simulink model "gm_uz_Deadbeat"  (R2022a)
settings: Solver=FixedStepDiscrete  StartTime=0.0  StopTime=10.0  RelTol=1e-3
settings Model: Creator=go98noz  LastModifiedBy=go98noz
settings SolverCC: AlgebraicLoopSolver=TrustRegion
settings DataIOCC: LimitDataPoints=on  SaveOutput=off  SaveTime=off
settings OptimizationCC: BlockReduction=off  ConditionallyExecuteInputs=off  DefaultParameterBehavior=Inlined  InheritOutputTypeSmallerThanSingle=on  LifeSpan=inf
settings DebuggingCC: AlgebraicLoopMsg=error  InheritedTsInSrcMsg=none  SingleTaskRateTransMsg=error  UnconnectedInputMsg=warning  UnconnectedOutputMsg=warning  UnconnectedLineMsg=warning  AllowSymbolicDim=off  StrictBusMsg=ErrorOnBusTreatedAsVector  SFUnexpectedBacktrackingDiag=warning  SFNoUnconditionalDefaultTransitionDiag=warning  SFExecutionAtInitializationDiag=none  SFMachineParentedDataDiag=warning  ArithmeticOperatorsInVariantConditions=warning
settings HardwareCC: ProdBitPerPointer=32  ProdBitPerSizeT=32  ProdBitPerPtrDiffT=32  ProdLargestAtomicFloat=None  ProdIntDivRoundTo=Undefined  ProdEndianess=Unspecified  ProdWordSize=32  ProdHWDeviceType=ASIC/FPGA->ASIC/FPGA  ProdEqTarget=off
settings SFSimCC: SimUseLocalCustomCode=off  CustomCodeUndefinedFunction=UseInterfaceOnly
settings RTWCC: RTWUseLocalCustomCode=off
settings CodeAppCC: StateflowObjectComments=on
settings GRTTargetCC: TargetLangStandard=C89/C90 (ANSI)
settings ConfigComp: CovScope=ReferencedModels  CovMetricSettings=dw  CovSaveCumulativeToWorkspaceVar=on  CovSaveSingleToWorkspaceVar=on  CovExternalEMLEnable=off  CovSFcnEnable=off

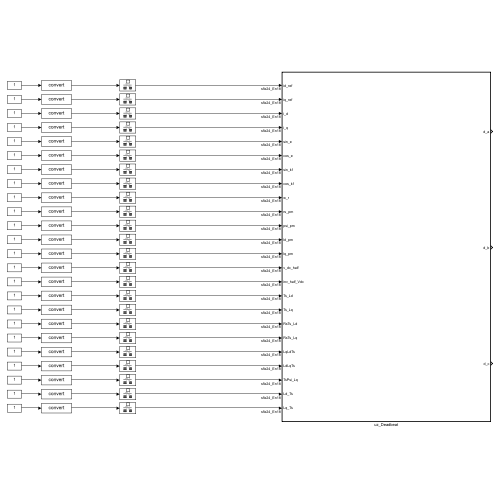
[thumbnail: Simulink's stored preview of the top-level diagram]
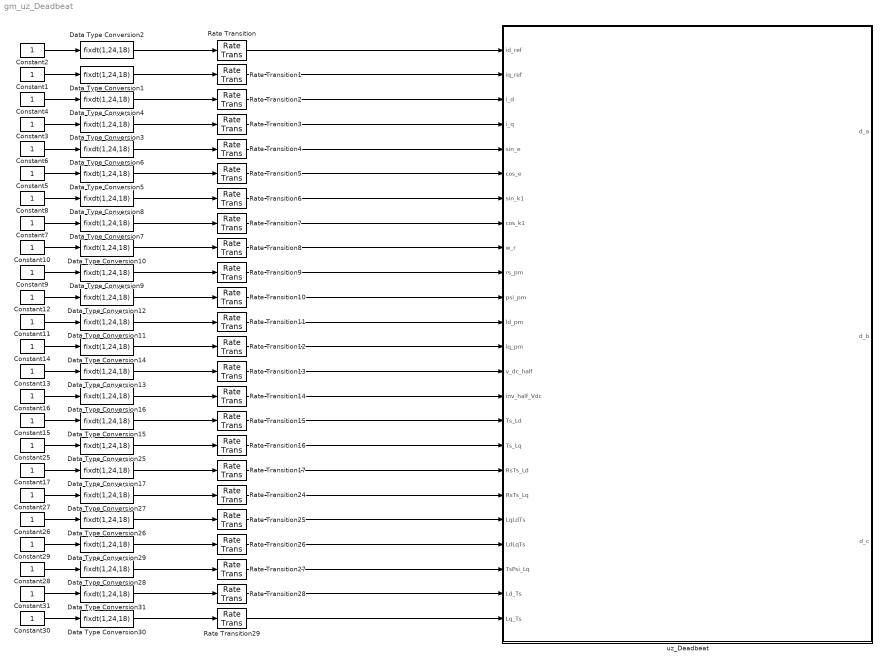
== system gm_uz_Deadbeat ==
  Constant{1..17,25..31} (24 alike) : Constant
  Data Type Conversion{1..17,25..31} (24 alike) : DataTypeConversion  OutDataTypeStr=fixdt(1,24,18)  SaturateOnIntegerOverflow=off  RndMeth=Floor
  Rate Transition{,1..17,24..29} (24 alike) : RateTransition  OutPortSampleTime=1/100e6
  uz_Deadbeat : Subsystem  TreatAsAtomicUnit=on
  wires:
  Rate Transition29/1 -> uz_Deadbeat/24(Lq_Ts)
  Rate Transition28/1 -> uz_Deadbeat/23(Ld_Ts)
  Rate Transition27/1 -> uz_Deadbeat/22(TsPsi_Lq)
  Rate Transition26/1 -> uz_Deadbeat/21(LdLqTs)
  Rate Transition25/1 -> uz_Deadbeat/20(LqLdTs)
  Rate Transition24/1 -> uz_Deadbeat/19(RsTs_Lq)
  Rate Transition17/1 -> uz_Deadbeat/18(RsTs_Ld)
  Rate Transition16/1 -> uz_Deadbeat/17(Ts_Lq)
  Rate Transition15/1 -> uz_Deadbeat/16(Ts_Ld)
  Rate Transition14/1 -> uz_Deadbeat/15(inv_half_Vdc)
  Rate Transition13/1 -> uz_Deadbeat/14(v_dc_half)
  Rate Transition12/1 -> uz_Deadbeat/13(lq_pm)
  Rate Transition11/1 -> uz_Deadbeat/12(ld_pm)
  Rate Transition10/1 -> uz_Deadbeat/11(psi_pm)
  Rate Transition9/1 -> uz_Deadbeat/10(rs_pm)
  Rate Transition8/1 -> uz_Deadbeat/9(w_r)
  Rate Transition7/1 -> uz_Deadbeat/8(cos_k1)
  Rate Transition6/1 -> uz_Deadbeat/7(sin_k1)
  Rate Transition5/1 -> uz_Deadbeat/6(cos_e)
  Rate Transition4/1 -> uz_Deadbeat/5(sin_e)
  Rate Transition3/1 -> uz_Deadbeat/4(i_q)
  Rate Transition2/1 -> uz_Deadbeat/3(i_d)
  Data Type Conversion17/1 -> Rate Transition17/1
  Constant17/1 -> Data Type Conversion17/1
  Constant25/1 -> Data Type Conversion25/1
  Data Type Conversion25/1 -> Rate Transition16/1
  Data Type Conversion27/1 -> Rate Transition24/1
  Constant27/1 -> Data Type Conversion27/1
  Constant26/1 -> Data Type Conversion26/1
  Data Type Conversion26/1 -> Rate Transition25/1
  Data Type Conversion30/1 -> Rate Transition29/1
  Constant30/1 -> Data Type Conversion30/1
  Constant31/1 -> Data Type Conversion31/1
  Data Type Conversion31/1 -> Rate Transition28/1
  Data Type Conversion29/1 -> Rate Transition26/1
  Constant29/1 -> Data Type Conversion29/1
  Constant28/1 -> Data Type Conversion28/1
  Data Type Conversion28/1 -> Rate Transition27/1
  Data Type Conversion9/1 -> Rate Transition9/1
  Constant9/1 -> Data Type Conversion9/1
  Constant10/1 -> Data Type Conversion10/1
  Data Type Conversion10/1 -> Rate Transition8/1
  Data Type Conversion12/1 -> Rate Transition10/1
  Constant12/1 -> Data Type Conversion12/1
  Constant11/1 -> Data Type Conversion11/1
  Data Type Conversion11/1 -> Rate Transition11/1
  Data Type Conversion15/1 -> Rate Transition15/1
  Constant15/1 -> Data Type Conversion15/1
  Constant16/1 -> Data Type Conversion16/1
  Data Type Conversion16/1 -> Rate Transition14/1
  Data Type Conversion14/1 -> Rate Transition12/1
  Constant14/1 -> Data Type Conversion14/1
  Constant13/1 -> Data Type Conversion13/1
  Data Type Conversion13/1 -> Rate Transition13/1
  Data Type Conversion5/1 -> Rate Transition5/1
  Constant5/1 -> Data Type Conversion5/1
  Constant6/1 -> Data Type Conversion6/1
  Data Type Conversion6/1 -> Rate Transition4/1
  Data Type Conversion8/1 -> Rate Transition6/1
  Constant8/1 -> Data Type Conversion8/1
  Constant7/1 -> Data Type Conversion7/1
  Data Type Conversion7/1 -> Rate Transition7/1
  Data Type Conversion3/1 -> Rate Transition3/1
  Constant3/1 -> Data Type Conversion3/1
  Constant4/1 -> Data Type Conversion4/1
  Data Type Conversion4/1 -> Rate Transition2/1
  Data Type Conversion2/1 -> Rate Transition/1
  Constant2/1 -> Data Type Conversion2/1
  Constant1/1 -> Data Type Conversion1/1
  Data Type Conversion1/1 -> Rate Transition1/1
  Rate Transition1/1 -> uz_Deadbeat/2(iq_ref)
  Rate Transition/1 -> uz_Deadbeat/1(id_ref)

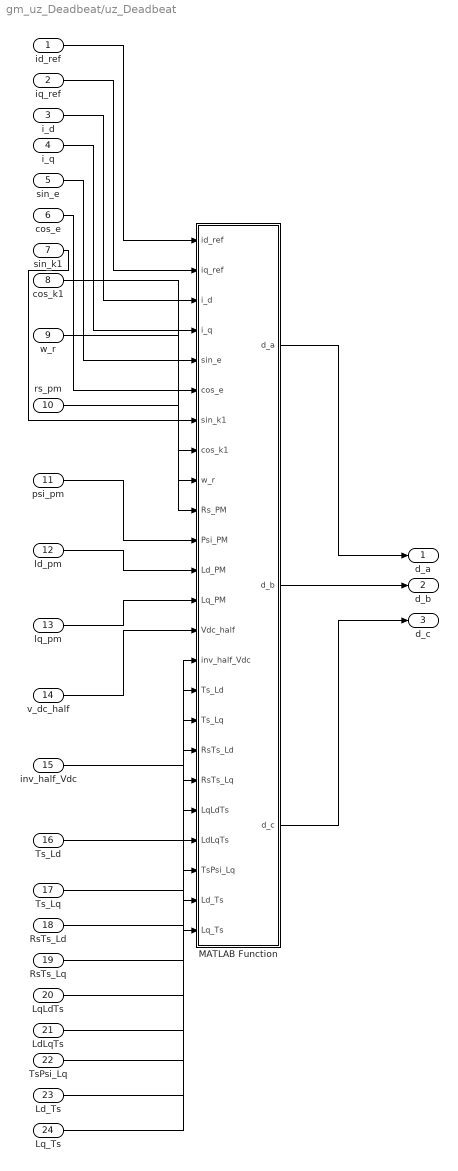
== system gm_uz_Deadbeat/uz_Deadbeat ==
  id_ref : Inport  OutDataTypeStr=fixdt(1, 24, 18)  PortDimensions=1  SampleTime=1e-08
  iq_ref : Inport  Port=2  OutDataTypeStr=fixdt(1, 24, 18)  PortDimensions=1  SampleTime=1e-08
  i_d : Inport  Port=3  OutDataTypeStr=fixdt(1, 24, 18)  PortDimensions=1  SampleTime=1e-08
  i_q : Inport  Port=4  OutDataTypeStr=fixdt(1, 24, 18)  PortDimensions=1  SampleTime=1e-08
  sin_e : Inport  Port=5  OutDataTypeStr=fixdt(1, 24, 18)  PortDimensions=1  SampleTime=1e-08
  cos_e : Inport  Port=6  OutDataTypeStr=fixdt(1, 24, 18)  PortDimensions=1  SampleTime=1e-08
  sin_k1 : Inport  Port=7  OutDataTypeStr=fixdt(1, 24, 18)  PortDimensions=1  SampleTime=1e-08
  cos_k1 : Inport  Port=8  OutDataTypeStr=fixdt(1, 24, 18)  PortDimensions=1  SampleTime=1e-08
  w_r : Inport  Port=9  OutDataTypeStr=fixdt(1, 24, 18)  PortDimensions=1  SampleTime=1e-08
  rs_pm : Inport  Port=10  OutDataTypeStr=fixdt(1, 24, 18)  PortDimensions=1  SampleTime=1e-08
  psi_pm : Inport  Port=11  OutDataTypeStr=fixdt(1, 24, 18)  PortDimensions=1  SampleTime=1e-08
  ld_pm : Inport  Port=12  OutDataTypeStr=fixdt(1, 24, 18)  PortDimensions=1  SampleTime=1e-08
  lq_pm : Inport  Port=13  OutDataTypeStr=fixdt(1, 24, 18)  PortDimensions=1  SampleTime=1e-08
  v_dc_half : Inport  Port=14  OutDataTypeStr=fixdt(1, 24, 18)  PortDimensions=1  SampleTime=1e-08
  inv_half_Vdc : Inport  Port=15  OutDataTypeStr=fixdt(1, 24, 18)  PortDimensions=1  SampleTime=1e-08
  Ts_Ld : Inport  Port=16  OutDataTypeStr=fixdt(1, 24, 18)  PortDimensions=1  SampleTime=1e-08
  Ts_Lq : Inport  Port=17  OutDataTypeStr=fixdt(1, 24, 18)  PortDimensions=1  SampleTime=1e-08
  RsTs_Ld : Inport  Port=18  OutDataTypeStr=fixdt(1, 24, 18)  PortDimensions=1  SampleTime=1e-08
  RsTs_Lq : Inport  Port=19  OutDataTypeStr=fixdt(1, 24, 18)  PortDimensions=1  SampleTime=1e-08
  LqLdTs : Inport  Port=20  OutDataTypeStr=fixdt(1, 24, 18)  PortDimensions=1  SampleTime=1e-08
  LdLqTs : Inport  Port=21  OutDataTypeStr=fixdt(1, 24, 18)  PortDimensions=1  SampleTime=1e-08
  TsPsi_Lq : Inport  Port=22  OutDataTypeStr=fixdt(1, 24, 18)  PortDimensions=1  SampleTime=1e-08
  Ld_Ts : Inport  Port=23  OutDataTypeStr=fixdt(1, 24, 18)  PortDimensions=1  SampleTime=1e-08
  Lq_Ts : Inport  Port=24  OutDataTypeStr=fixdt(1, 24, 18)  PortDimensions=1  SampleTime=1e-08
  MATLAB Function : Subsystem
  d_a : Outport  SampleTime=1e-08  VectorParamsAs1DForOutWhenUnconnected=off
  d_b : Outport  Port=2  SampleTime=1e-08  VectorParamsAs1DForOutWhenUnconnected=off
  d_c : Outport  Port=3  SampleTime=1e-08  VectorParamsAs1DForOutWhenUnconnected=off
  wires:
  id_ref/1 -> MATLAB Function/1(id_ref)
  iq_ref/1 -> MATLAB Function/2(iq_ref)
  i_d/1 -> MATLAB Function/3(i_d)
  i_q/1 -> MATLAB Function/4(i_q)
  sin_e/1 -> MATLAB Function/5(sin_e)
  cos_e/1 -> MATLAB Function/6(cos_e)
  sin_k1/1 -> MATLAB Function/7(sin_k1)
  cos_k1/1 -> MATLAB Function/8(cos_k1)
  w_r/1 -> MATLAB Function/9(w_r)
  rs_pm/1 -> MATLAB Function/10(Rs_PM)
  psi_pm/1 -> MATLAB Function/11(Psi_PM)
  ld_pm/1 -> MATLAB Function/12(Ld_PM)
  lq_pm/1 -> MATLAB Function/13(Lq_PM)
  v_dc_half/1 -> MATLAB Function/14(Vdc_half)
  inv_half_Vdc/1 -> MATLAB Function/15(inv_half_Vdc)
  Ts_Ld/1 -> MATLAB Function/16(Ts_Ld)
  Ts_Lq/1 -> MATLAB Function/17(Ts_Lq)
  RsTs_Ld/1 -> MATLAB Function/18(RsTs_Ld)
  RsTs_Lq/1 -> MATLAB Function/19(RsTs_Lq)
  LqLdTs/1 -> MATLAB Function/20(LqLdTs)
  LdLqTs/1 -> MATLAB Function/21(LdLqTs)
  TsPsi_Lq/1 -> MATLAB Function/22(TsPsi_Lq)
  Ld_Ts/1 -> MATLAB Function/23(Ld_Ts)
  Lq_Ts/1 -> MATLAB Function/24(Lq_Ts)
  MATLAB Function/1(d_a) -> d_a/1
  MATLAB Function/2(d_b) -> d_b/1
  MATLAB Function/3(d_c) -> d_c/1

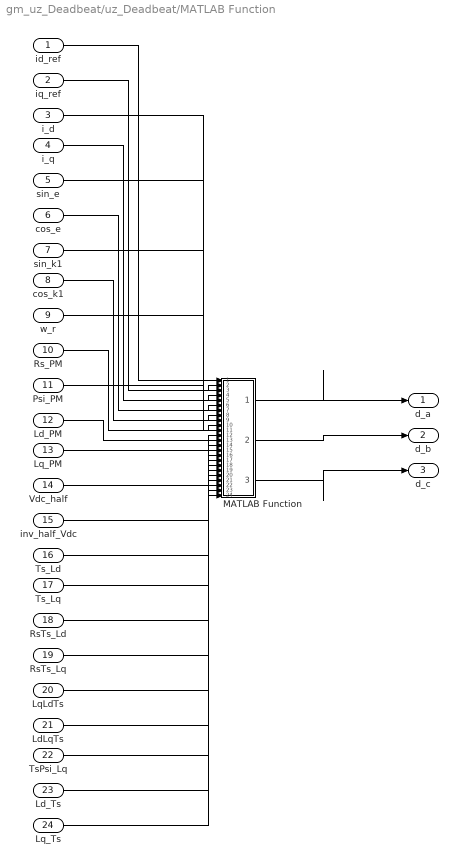
== system gm_uz_Deadbeat/uz_Deadbeat/MATLAB Function ==
  id_ref : Inport  OutDataTypeStr=fixdt(1, 24, 18)  PortDimensions=1  SampleTime=1e-08
  iq_ref : Inport  Port=2  OutDataTypeStr=fixdt(1, 24, 18)  PortDimensions=1  SampleTime=1e-08
  i_d : Inport  Port=3  OutDataTypeStr=fixdt(1, 24, 18)  PortDimensions=1  SampleTime=1e-08
  i_q : Inport  Port=4  OutDataTypeStr=fixdt(1, 24, 18)  PortDimensions=1  SampleTime=1e-08
  sin_e : Inport  Port=5  OutDataTypeStr=fixdt(1, 24, 18)  PortDimensions=1  SampleTime=1e-08
  cos_e : Inport  Port=6  OutDataTypeStr=fixdt(1, 24, 18)  PortDimensions=1  SampleTime=1e-08
  sin_k1 : Inport  Port=7  OutDataTypeStr=fixdt(1, 24, 18)  PortDimensions=1  SampleTime=1e-08
  cos_k1 : Inport  Port=8  OutDataTypeStr=fixdt(1, 24, 18)  PortDimensions=1  SampleTime=1e-08
  w_r : Inport  Port=9  OutDataTypeStr=fixdt(1, 24, 18)  PortDimensions=1  SampleTime=1e-08
  Rs_PM : Inport  Port=10  OutDataTypeStr=fixdt(1, 24, 18)  PortDimensions=1  SampleTime=1e-08
  Psi_PM : Inport  Port=11  OutDataTypeStr=fixdt(1, 24, 18)  PortDimensions=1  SampleTime=1e-08
  Ld_PM : Inport  Port=12  OutDataTypeStr=fixdt(1, 24, 18)  PortDimensions=1  SampleTime=1e-08
  Lq_PM : Inport  Port=13  OutDataTypeStr=fixdt(1, 24, 18)  PortDimensions=1  SampleTime=1e-08
  Vdc_half : Inport  Port=14  OutDataTypeStr=fixdt(1, 24, 18)  PortDimensions=1  SampleTime=1e-08
  inv_half_Vdc : Inport  Port=15  OutDataTypeStr=fixdt(1, 24, 18)  PortDimensions=1  SampleTime=1e-08
  Ts_Ld : Inport  Port=16  OutDataTypeStr=fixdt(1, 24, 18)  PortDimensions=1  SampleTime=1e-08
  Ts_Lq : Inport  Port=17  OutDataTypeStr=fixdt(1, 24, 18)  PortDimensions=1  SampleTime=1e-08
  RsTs_Ld : Inport  Port=18  OutDataTypeStr=fixdt(1, 24, 18)  PortDimensions=1  SampleTime=1e-08
  RsTs_Lq : Inport  Port=19  OutDataTypeStr=fixdt(1, 24, 18)  PortDimensions=1  SampleTime=1e-08
  LqLdTs : Inport  Port=20  OutDataTypeStr=fixdt(1, 24, 18)  PortDimensions=1  SampleTime=1e-08
  LdLqTs : Inport  Port=21  OutDataTypeStr=fixdt(1, 24, 18)  PortDimensions=1  SampleTime=1e-08
  TsPsi_Lq : Inport  Port=22  OutDataTypeStr=fixdt(1, 24, 18)  PortDimensions=1  SampleTime=1e-08
  Ld_Ts : Inport  Port=23  OutDataTypeStr=fixdt(1, 24, 18)  PortDimensions=1  SampleTime=1e-08
  Lq_Ts : Inport  Port=24  OutDataTypeStr=fixdt(1, 24, 18)  PortDimensions=1  SampleTime=1e-08
  MATLAB Function : MATLAB Function  TreatAsAtomicUnit=on
  d_a : Outport  SampleTime=1e-08  VectorParamsAs1DForOutWhenUnconnected=off
  d_b : Outport  Port=2  SampleTime=1e-08
  d_c : Outport  Port=3  SampleTime=1e-08
  wires:
  id_ref/1 -> MATLAB Function/1(id_ref)
  iq_ref/1 -> MATLAB Function/2(iq_ref)
  i_d/1 -> MATLAB Function/3(i_d)
  i_q/1 -> MATLAB Function/4(i_q)
  sin_e/1 -> MATLAB Function/5(sin_e)
  cos_e/1 -> MATLAB Function/6(cos_e)
  sin_k1/1 -> MATLAB Function/7(sin_k1)
  cos_k1/1 -> MATLAB Function/8(cos_k1)
  w_r/1 -> MATLAB Function/9(w_r)
  Rs_PM/1 -> MATLAB Function/10(Rs_PM)
  Psi_PM/1 -> MATLAB Function/11(Psi_PM)
  Ld_PM/1 -> MATLAB Function/12(Ld_PM)
  Lq_PM/1 -> MATLAB Function/13(Lq_PM)
  Vdc_half/1 -> MATLAB Function/14(Vdc_half)
  inv_half_Vdc/1 -> MATLAB Function/15(inv_half_Vdc)
  Ts_Ld/1 -> MATLAB Function/16(Ts_Ld)
  Ts_Lq/1 -> MATLAB Function/17(Ts_Lq)
  RsTs_Ld/1 -> MATLAB Function/18(RsTs_Ld)
  RsTs_Lq/1 -> MATLAB Function/19(RsTs_Lq)
  LqLdTs/1 -> MATLAB Function/20(LqLdTs)
  LdLqTs/1 -> MATLAB Function/21(LdLqTs)
  TsPsi_Lq/1 -> MATLAB Function/22(TsPsi_Lq)
  Ld_Ts/1 -> MATLAB Function/23(Ld_Ts)
  Lq_Ts/1 -> MATLAB Function/24(Lq_Ts)
  MATLAB Function/1(d_a) -> d_a/1
  MATLAB Function/2(d_b) -> d_b/1
  MATLAB Function/3(d_c) -> d_c/1

== matlab function gm_uz_Deadbeat/uz_Deadbeat/MATLAB Function/MATLAB Function ==
  settings: fimath=fimath('RoundingMethod', 'Floor','OverflowAction', 'Wrap','ProductMode', 'FullPrecision', 'SumMode', 'FullPrecision')
  data: id_ref input; d_a output fixdt(0,16,15); iq_ref input; i_d input; i_q input; sin_e input; cos_e input; sin_k1 input; cos_k1 input; w_r input; Rs_PM input; Psi_PM input; Ld_PM input; Lq_PM input; Vdc_half input; inv_half_Vdc input; Ts_Ld input; d_b output fixdt(0,16,15); d_c output fixdt(0,16,15); Ts_Lq input; RsTs_Ld input; RsTs_Lq input; LqLdTs input; LdLqTs input; TsPsi_Lq input; Ld_Ts input; Lq_Ts input
function [d_a, d_b, d_c] = DB_PWM( ...
    id_ref, iq_ref, i_d, i_q, ...
    sin_e, cos_e, sin_k1, cos_k1, ...
    w_r, Rs_PM, Psi_PM, Ld_PM, Lq_PM, ...
    Vdc_half, inv_half_Vdc, ...
    Ts_Ld, Ts_Lq, RsTs_Ld, RsTs_Lq, ...
    LqLdTs, LdLqTs, TsPsi_Lq, ...
    Ld_Ts, Lq_Ts)

%#codegen

Tcur  = numerictype(1,24,16);
Tvol  = numerictype(1,24,10);
Tmod  = numerictype(1,18,16);
Tcoef = numerictype(1,24,18);
Ttrig = numerictype(1,18,16);
Tout  = numerictype(0,16,15);

F = fimath( ...
    'RoundingMethod','Nearest', ...
    'OverflowAction','Saturate', ...
    'ProductMode','SpecifyPrecision', ...
    'ProductWordLength',32, ...
    'ProductFractionLength',20, ...
    'SumMode','SpecifyPrecision', ...
    'SumWordLength',32, ...
    'SumFractionLength',20);

id_ref = fi(id_ref, Tcur, F);
iq_ref = fi(iq_ref, Tcur, F);
i_d    = fi(i_d,    Tcur, F);
i_q    = fi(i_q,    Tcur, F);

sin_e  = fi(sin_e,  Ttrig, F);
cos_e  = fi(cos_e,  Ttrig, F);
sin_k1 = fi(sin_k1, Ttrig, F);
cos_k1 = fi(cos_k1, Ttrig, F);

w_r          = fi(w_r,          Tcoef, F);
Rs_PM        = fi(Rs_PM,        Tcoef, F);
Psi_PM       = fi(Psi_PM,       Tcoef, F);
Ld_PM        = fi(Ld_PM,        Tcoef, F);
Lq_PM        = fi(Lq_PM,        Tcoef, F);
Vdc_half     = fi(Vdc_half,     Tcoef, F);
inv_half_Vdc = fi(inv_half_Vdc, Tcoef, F);

Ts_Ld     = fi(Ts_Ld,     Tcoef, F);
Ts_Lq     = fi(Ts_Lq,     Tcoef, F);
RsTs_Ld   = fi(RsTs_Ld,   Tcoef, F);
RsTs_Lq   = fi(RsTs_Lq,   Tcoef, F);
LqLdTs    = fi(LqLdTs,    Tcoef, F);
LdLqTs    = fi(LdLqTs,    Tcoef, F);
TsPsi_Lq  = fi(TsPsi_Lq,  Tcoef, F);
Ld_Ts     = fi(Ld_Ts,     Tcoef, F);
Lq_Ts     = fi(Lq_Ts,     Tcoef, F);

zero_mod = fi(0, Tmod, F);

persistent u_a0 u_b0 u_c0;
if isempty(u_a0)
    u_a0 = zero_mod;
    u_b0 = zero_mod;
    u_c0 = zero_mod;
end

[u_alpha0, u_beta0] = T_C(u_a0, u_b0, u_c0, F);

[u_d0, u_q0] = T_P(u_alpha0, u_beta0, sin_e, cos_e, F);

v_d0 = fi(u_d0 * Vdc_half, Tvol, F);
v_q0 = fi(u_q0 * Vdc_half, Tvol, F);

one_coef = fi(1, Tcoef, F);

term_id1 = fi(Ts_Ld * v_d0, Tcur, F);
term_id2 = fi(fi(one_coef - RsTs_Ld, Tcoef, F) * i_d, Tcur, F);
term_id3 = fi(fi(LqLdTs * w_r, Tcoef, F) * i_q, Tcur, F);

id_k = fi(term_id1 + term_id2 + term_id3, Tcur, F);

term_iq1 = fi(Ts_Lq * v_q0, Tcur, F);
term_iq2 = fi(fi(one_coef - RsTs_Lq, Tcoef, F) * i_q, Tcur, F);
term_iq3 = fi(fi(LdLqTs * w_r, Tcoef, F) * i_d, Tcur, F);
term_iq4 = fi(TsPsi_Lq * w_r, Tcur, F);

iq_k = fi(term_iq1 + term_iq2 - term_iq3 - term_iq4, Tcur, F);

err_d = fi(id_ref - id_k, Tcur, F);
err_q = fi(iq_ref - iq_k, Tcur, F);

term_vd1 = fi(Ld_Ts * err_d, Tvol, F);
term_vd2 = fi(Rs_PM * id_k,  Tvol, F);
term_vd3 = fi(fi(Lq_PM * w_r, Tcoef, F) * iq_k, Tvol, F);

vd_ref = fi(term_vd1 + term_vd2 - term_vd3, Tvol, F);

term_vq1 = fi(Lq_Ts * err_q, Tvol, F);
term_vq2 = fi(Rs_PM * iq_k,  Tvol, F);
term_vq3 = fi(fi(Ld_PM * w_r, Tcoef, F) * id_k, Tvol, F);
term_vq4 = fi(w_r * Psi_PM, Tvol, F);

vq_ref = fi(term_vq1 + term_vq2 + term_vq3 + term_vq4, Tvol, F);

[v_alpha_ref, v_beta_ref] = T_P_inv(vd_ref, vq_ref, sin_k1, cos_k1, F);

u_alpha = fi(v_alpha_ref * inv_half_Vdc, Tmod, F);
u_beta  = fi(v_beta_ref  * inv_half_Vdc, Tmod, F);

[u_a, u_b, u_c] = T_C_inv(u_alpha, u_beta, F);

u_min = min3(u_a, u_b, u_c);
u_max = max3(u_a, u_b, u_c);

u_com = fi(fi(-0.5, Tmod, F) * fi(u_min + u_max, Tmod, F), Tmod, F);

u_a = fi(u_a + u_com, Tmod, F);
u_b = fi(u_b + u_com, Tmod, F);
u_c = fi(u_c + u_com, Tmod, F);

u_a = sat_pm1(u_a, F);
u_b = sat_pm1(u_b, F);
u_c = sat_pm1(u_c, F);

d_a = fi((u_a + fi(1, Tmod, F)) * fi(0.5, Tmod, F), Tout, F);
d_b = fi((u_b + fi(1, Tmod, F)) * fi(0.5, Tmod, F), Tout, F);
d_c = fi((u_c + fi(1, Tmod, F)) * fi(0.5, Tmod, F), Tout, F);

u_a0 = u_a;
u_b0 = u_b;
u_c0 = u_c;

end


function [alpha, beta] = T_C(a, b, c, F)

Tmod = numerictype(1,18,16);

k1 = fi(0.6666666666666667, Tmod, F);
k2 = fi(0.5,                Tmod, F);
k3 = fi(0.5773502691896258, Tmod, F);

tmp_alpha = fi(a - k2*b - k2*c, Tmod, F);
alpha = fi(k1 * tmp_alpha, Tmod, F);

tmp_beta = fi(b - c, Tmod, F);
beta = fi(k3 * tmp_beta, Tmod, F);

end


function [d, q] = T_P(alpha, beta, sinTheta, cosTheta, F)

Tmod = numerictype(1,18,16);

d = fi(fi(cosTheta * alpha, Tmod, F) + fi(sinTheta * beta, Tmod, F), Tmod, F);
q = fi(fi(-sinTheta * alpha, Tmod, F) + fi(cosTheta * beta, Tmod, F), Tmod, F);

end


function [alpha, beta] = T_P_inv(d, q, sinTheta, cosTheta, F)

Tvol = numerictype(1,24,10);

alpha = fi(fi(cosTheta * d, Tvol, F) - fi(sinTheta * q, Tvol, F), Tvol, F);
beta  = fi(fi(sinTheta * d, Tvol, F) + fi(cosTheta * q, Tvol, F), Tvol, F);

end


function [a, b, c] = T_C_inv(alpha, beta, F)

Tmod = numerictype(1,18,16);

k1 = fi(-0.5,               Tmod, F);
k2 = fi(0.8660254037844386, Tmod, F);

a = fi(alpha, Tmod, F);
b = fi(k1*alpha + k2*beta, Tmod, F);
c = fi(k1*alpha - k2*beta, Tmod, F);

end


function y = sat_pm1(x, F)

Tmod = numerictype(1,18,16);

one  = fi(1,  Tmod, F);
none = fi(-1, Tmod, F);

if x > one
    y = one;
elseif x < none
    y = none;
else
    y = fi(x, Tmod, F);
end

end


function y = min3(a, b, c)

y = a;

if b < y
    y = b;
end

if c < y
    y = c;
end

end


function y = max3(a, b, c)

y = a;

if b > y
    y = b;
end

if c > y
    y = c;
end

end
